simulink model "maths"  (R2024b)
settings: Solver=VariableStepAuto  StartTime=0.0  StopTime=10.0  RelTol=1e-3
libraries: fl_lib x20
settings Model: Creator=manoharpaturi  LastModifiedBy=manoharpaturi

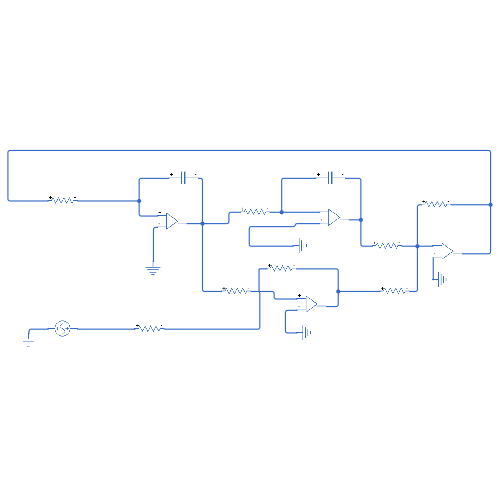
[thumbnail: Simulink's stored preview of the top-level diagram]
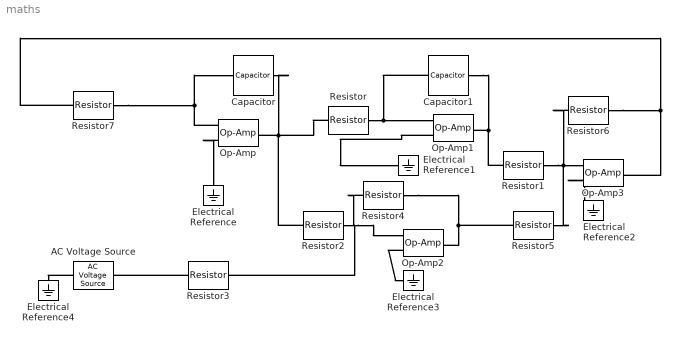
== system maths ==
  AC Voltage Source : fl_lib/Electrical/Electrical Sources/AC Voltage Source  amp=1 V  shift=0 deg  frequency=60 Hz
  Capacitor : fl_lib/Electrical/Electrical Elements/Capacitor  c=1e-6 F  r=1e-6 Ohm  g=0 1/Ohm  i_specify=off  i_priority=None  i=0 A  i_nominal_specify=off  i_nominal_value=1  i_nominal_unit=A  v_specify=off  v_priority=None  v=0 V  v_nominal_specify=off  v_nominal_value=1  v_nominal_unit=V  vc_specify=off  vc_priority=High  vc=0 V  vc_nominal_specify=off  vc_nominal_value=1  vc_nominal_unit=V
  Capacitor1 : fl_lib/Electrical/Electrical Elements/Capacitor  c=1e-6 F  r=1e-6 Ohm  g=0 1/Ohm  i_specify=off  i_priority=None  i=0 A  i_nominal_specify=off  i_nominal_value=1  i_nominal_unit=A  v_specify=off  v_priority=None  v=0 V  v_nominal_specify=off  v_nominal_value=1  v_nominal_unit=V  vc_specify=off  vc_priority=High  vc=0 V  vc_nominal_specify=off  vc_nominal_value=1  vc_nominal_unit=V
  Electrical Reference{,1..4} (5 alike) : fl_lib/Electrical/Electrical Elements/Electrical Reference
  Op-Amp{,1..3} (4 alike) : fl_lib/Electrical/Electrical Elements/Op-Amp  outI_specify=off  outI_priority=None  outI=0 A  outI_nominal_specify=off  outI_nominal_value=1  outI_nominal_unit=A
  Resistor{,1..7} (8 alike) : fl_lib/Electrical/Electrical Elements/Resistor  R=1 Ohm  i_specify=off  i_priority=None  i=0 A  i_nominal_specify=off  i_nominal_value=1  i_nominal_unit=A  v_specify=off  v_priority=None  v=0 V  v_nominal_specify=off  v_nominal_value=1  v_nominal_unit=V
  connections:
  Op-Amp/LConn1 -- Resistor7/RConn1 -- Capacitor/LConn1
  Capacitor/RConn1 -- Resistor2/LConn1 -- Resistor/LConn1 -- Op-Amp/RConn1
  Resistor/RConn1 -- Capacitor1/LConn1 -- Op-Amp1/LConn1
  Capacitor1/RConn1 -- Resistor1/LConn1 -- Op-Amp1/RConn1
  Resistor1/RConn1 -- Resistor6/LConn1 -- Resistor5/RConn1 -- Op-Amp3/LConn1
  Op-Amp/LConn2 -- Electrical Reference/LConn1
  Op-Amp1/LConn2 -- Electrical Reference1/LConn1
  Op-Amp3/LConn2 -- Electrical Reference2/LConn1
  Resistor2/RConn1 -- Op-Amp2/LConn1
  Resistor4/RConn1 -- Op-Amp2/RConn1 -- Resistor5/LConn1
  Op-Amp2/LConn2 -- Electrical Reference3/LConn1
  Resistor6/RConn1 -- Op-Amp3/RConn1 -- Resistor7/LConn1
  Resistor3/LConn1 -- AC Voltage Source/LConn1
  AC Voltage Source/RConn1 -- Electrical Reference4/LConn1
  Resistor4/LConn1 -- Resistor3/RConn1
